simulink model "model_v0"  (R2020b)
settings: Solver=VariableStepAuto  StartTime=15  StopTime=30  RelTol=1e-3
settings Model: Creator=a1  LastModifiedBy=a1
settings HardwareCC: ProdBitPerLong=64  ProdHWDeviceType=Intel->x86-64 (Mac OS X)

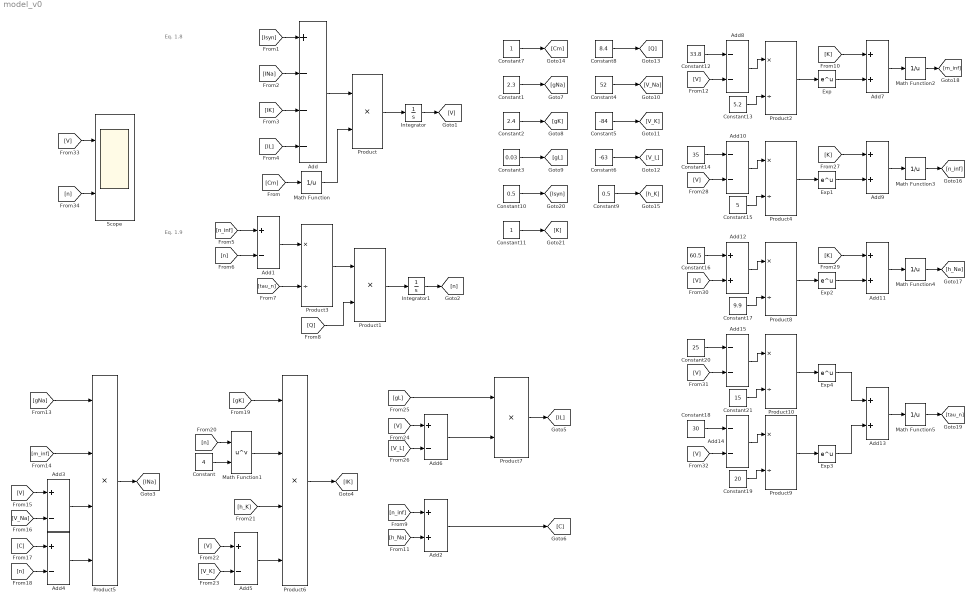
== system model_v0 ==
  note: Eq. 1.8
  note: Eq. 1.9
  Add : Sum  Inputs=+---
  Add{1,3..6} (5 alike) : Sum  Inputs=+-
  Add{8,10,14..15} (4 alike) : Sum  Inputs=--
  Add{2,7,9,11..13} (6 alike) : Sum
  Constant : Constant  Value=4
  Constant1 : Constant  Value=2.3
  Constant10 : Constant  Value=0.5
  Constant11 : Constant
  Constant12 : Constant  Value=33.8
  Constant13 : Constant  Value=5.2
  Constant14 : Constant  Value=35
  Constant15 : Constant  Value=5
  Constant16 : Constant  Value=60.5
  Constant17 : Constant  Value=9.9
  Constant18 : Constant  Value=30
  Constant19 : Constant  Value=20
  Constant2 : Constant  Value=2.4
  Constant20 : Constant  Value=25
  Constant21 : Constant  Value=15
  Constant3 : Constant  Value=0.03
  Constant4 : Constant  Value=52
  Constant5 : Constant  Value=-84
  Constant6 : Constant  Value=-63
  Constant7 : Constant
  Constant8 : Constant  Value=8.4
  Constant9 : Constant  Value=0.5
  Exp{,1..4} (5 alike) : Math  SaturateOnIntegerOverflow=on
  Integrator : Integrator
  Integrator1 : Integrator
  Math Function{,2..5} (5 alike) : Math  Operator=reciprocal  SignedPower=on  SaturateOnIntegerOverflow=on
  Math Function1 : Math  Operator=pow  SignedPower=on  SaturateOnIntegerOverflow=on
  Product : Product
  Product1 : Product
  Product{2..4,8..10} (6 alike) : Product  Inputs=*/
  Product5 : Product  Inputs=4
  Product6 : Product  Inputs=4
  Product7 : Product
  Scope : Scope  NumInputPorts=2
  wires:
  [INa] -> Add/2
  Math Function/1 -> Product/2
  Add/1 -> Product/1
  [Isyn] -> Add/1
  Product/1 -> Integrator/1
  [IL] -> Add/4
  [Cm] -> Math Function/1
  Integrator/1 -> [V]
  Add1/1 -> Product3/1
  [n_inf] -> Add1/1
  [tau_n] -> Product3/2
  [n] -> Add1/2
  Product3/1 -> Product1/1
  Integrator1/1 -> [n]
  Product1/1 -> Integrator1/1
  [IK] -> Add/3
  [Q] -> Product1/2
  Add3/1 -> Product5/3
  [C] -> Add4/1
  [V] -> Add3/1
  Product5/1 -> [INa]
  [m_inf] -> Product5/2
  [gNa] -> Product5/1
  Add4/1 -> Product5/4
  [V_Na] -> Add3/2
  [n] -> Add4/2
  [V_K] -> Add5/2
  [V] -> Add5/1
  Constant/1 -> Math Function1/2
  [n] -> Math Function1/1
  Add5/1 -> Product6/4
  [h_K] -> Product6/3
  Math Function1/1 -> Product6/2
  [gK] -> Product6/1
  Product6/1 -> [IK]
  [V_L] -> Add6/2
  [V] -> Add6/1
  Add6/1 -> Product7/2
  [gL] -> Product7/1
  Product7/1 -> [IL]
  [h_Na] -> Add2/2
  Add2/1 -> [C]
  [n_inf] -> Add2/1
  Constant3/1 -> [gL]
  Constant1/1 -> [gNa]
  Constant2/1 -> [gK]
  Constant4/1 -> [V_Na]
  Constant5/1 -> [V_K]
  Constant6/1 -> [V_L]
  Constant8/1 -> [Q]
  Constant7/1 -> [Cm]
  Constant9/1 -> [h_K]
  Constant10/1 -> [Isyn]
  [K] -> Add7/1
  Constant11/1 -> [K]
  Constant12/1 -> Add8/1
  [V] -> Add8/2
  Add8/1 -> Product2/1
  Constant13/1 -> Product2/2
  Product2/1 -> Exp/1
  Exp/1 -> Add7/2
  Add7/1 -> Math Function2/1
  [K] -> Add9/1
  Math Function3/1 -> [n_inf]
  Add10/1 -> Product4/1
  [V] -> Add10/2
  Constant15/1 -> Product4/2
  Constant14/1 -> Add10/1
  Product4/1 -> Exp1/1
  Add9/1 -> Math Function3/1
  Exp1/1 -> Add9/2
  [K] -> Add11/1
  Add12/1 -> Product8/1
  [V] -> Add12/2
  Constant17/1 -> Product8/2
  Constant16/1 -> Add12/1
  Product8/1 -> Exp2/1
  Add11/1 -> Math Function4/1
  Exp2/1 -> Add11/2
  Add14/1 -> Product9/1
  [V] -> Add14/2
  Constant19/1 -> Product9/2
  Constant18/1 -> Add14/1
  Product9/1 -> Exp3/1
  Add13/1 -> Math Function5/1
  Exp3/1 -> Add13/2
  Math Function2/1 -> [m_inf]
  Math Function4/1 -> [h_Na]
  Math Function5/1 -> [tau_n]
  Add15/1 -> Product10/1
  Constant20/1 -> Add15/1
  [V] -> Add15/2
  Product10/1 -> Exp4/1
  Constant21/1 -> Product10/2
  Exp4/1 -> Add13/1
  [V] -> Scope/1
  [n] -> Scope/2
